simulink model "NewMY"  (Simulink 7.8)
settings: Solver=ode45  StartTime=0.0  StopTime=6  RelTol=1e-3
undefined symbols (not defined in the file): DiscIntNeverNeededParam
libraries: powerlib x8, simulink x4, powerlib_extras x2
settings Model: Creator=Meshkov  LastModifiedBy=suzdorf.vi  ModifiedComment=Meshkov -- Fri Mar 25 16:39:32 2011 -- Version 1.11
settings Model: ModifiedHistory=|
  | Meshkov -- Fri Mar 25 16:39:32 2011 -- Version 1.11
  | 
  | 
  | Meshkov -- Fri Mar 25 12:43:29 2011 -- Version 1.10
  | 
  | 
  | Meshkov -- Thu Mar 03 20:00:01 2011 -- Version 1.9
  | 
  | 
  | Meshkov -- Thu Mar 03 18:37:37 2011 -- Version 1.8
  | 
  | 
  | This model was created by Aleksander S. Meshkov on Feb 28. I don't khiw why I created that model...
  | so... may be i had wanted to write dissertation
settings DataIOCC: LimitDataPoints=off
settings DebuggingCC: FcnCallInpInsideContextMsg=Use local settings

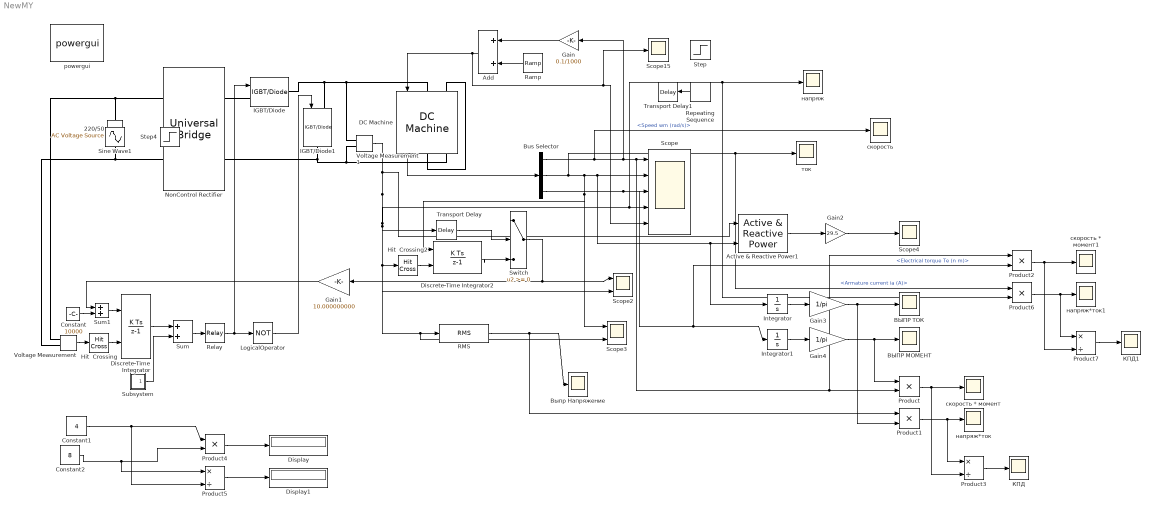
== system NewMY ==
  220/50 : powerlib/Electrical Sources/AC Voltage Source  Amplitude=220*sqrt(2)  Phase=0  Frequency=50  SampleTime=0  Measurements=None
  Active & Reactive Power1 : powerlib_extras/Measurements/Active & Reactive Power  f1=100
  Add : Sum
  Bus Selector : BusSelector  OutputSignals=Speed wm (rad/s),Armature current ia (A),Electrical torque Te (n m)
  Constant : Constant  Value=10000  SampleTime=0
  Constant1 : Constant  Value=4
  Constant2 : Constant  Value=8
  DC Machine : powerlib/Machines/DC Machine  PresetModel=No  MechanicalLoad=Torque TL  FieldType=Wound  ShowDetailedParameters=on  RLa="[ 7.061  0.058]"  RLf="[ 12.939  0.531]"  Laf=0.0098  MachineConstant=Torque constant (N.m/A)  Ke=1.8  Kt=1.8  J=0.21e-3  Bm=0  Tf=0  w0=1  Ifinit=-8.46539071434242e-022  TsPowergui=0  TsBlock=-1
      settings: AttributesFormatString=\n
  Discrete-Time Integrator : DiscreteIntegrator  gainval=1  ExternalReset=rising  SampleTime=2e-005  ICPrevOutput=DiscIntNeverNeededParam  ICPrevScaledInput=DiscIntNeverNeededParam
  Discrete-Time Integrator2 : DiscreteIntegrator  gainval=1  ExternalReset=rising  SampleTime=2e-005  ICPrevOutput=DiscIntNeverNeededParam  ICPrevScaledInput=DiscIntNeverNeededParam
  Display : Display
  Display1 : Display
  Gain : Gain  Gain=0.1/1000
  Gain1 : Gain  Gain=10.000000000
  Gain2 : Gain  Gain=29.5
  Gain3 : Gain  Gain=1/pi
  Gain4 : Gain  Gain=1/pi
  Hit  Crossing : HitCross  SampleTime=2e-005
  Hit  Crossing2 : HitCross  SampleTime=2e-005
  IGBT/Diode : powerlib/Power Electronics/IGBT//Diode  Ron=1e-3  Rs=1e5  Cs=inf  Measurements=off
  IGBT/Diode1 : powerlib/Power Electronics/IGBT//Diode  Ron=1e-3  Rs=1e5  Cs=inf  Measurements=off
  Integrator : Integrator
  Integrator1 : Integrator
  LogicalOperator : Logic  Operator=NOT  AllPortsSameDT=off  OutDataTypeStr=boolean
  NonControl Rectifier : powerlib/Power Electronics/Universal Bridge  Arms=2  SnubberResistance=1e5  SnubberCapacitance=inf  Device=Diodes  Ron=1e-3  Lon=0  ForwardVoltages="[  0  0  ]"  ForwardVoltage=0  GTOparameters=[ 10e-6 , 20e-6 ]  IGBTparameters=[ 1e-6 , 2e-6 ]  Measurements=Device currents  Measurements_2=None  converterType=Rectifier
  Product{,1..2,4,6} (5 alike) : Product  RndMeth=Zero
  Product3 : Product  Inputs=*/  RndMeth=Zero
  Product5 : Product  Inputs=*/  SaturateOnIntegerOverflow=on  RndMeth=Zero
  Product7 : Product  Inputs=*/  RndMeth=Zero
  RMS : powerlib_extras/Measurements/RMS  f1=100
  Ramp : simulink/Sources/Ramp  slope=-0.2  start=3  X0=0
  Relay : Relay  OnSwitchValue=0.1  OffSwitchValue=-0.1  OutDataTypeStr=Inherit: Inherit via back propagation
  Repeating Sequence : simulink/Sources/Repeating Sequence  rep_seq_t=[0 1]  rep_seq_y=[0 0.35]
  Scope : Scope  NumInputPorts=5
      settings: YMin=649.5~7.1~0.49~-50~0.5818  YMax=652~7.9~0.61~350~0.5827
  Scope15 : Scope
      settings: YMin=0  YMax=0.02  SaveName=Mc
  Scope2 : Scope  NumInputPorts=2
      settings: YMin=0~0  YMax=0.02~1  SaveName=current
  Scope3 : Scope  NumInputPorts=2
      settings: YMin=0~0  YMax=0.02~1  SaveName=current1
  Scope4 : Scope
      settings: YMin=0  YMax=0.02  SaveName=Mc1
  Step : Step  Time=4  After=0.252  SampleTime=0
  Subsystem : Subsystem
      mask Display: port_label('output', 1, '-C-')
  Sum : Sum  SaturateOnIntegerOverflow=on  InputSameDT=on  OutDataTypeStr=Inherit: Same as first input
  Sum1 : Sum  SaturateOnIntegerOverflow=on  InputSameDT=on  OutDataTypeStr=Inherit: Same as first input
  Switch : Switch  OutDataTypeStr=double  ZeroCross=off
  Transport Delay : TransportDelay  DelayTime=0.00003
  Transport Delay1 : TransportDelay  DelayTime=3
  Voltage Measurement : powerlib/Measurements/Voltage Measurement  PhasorSimulation=off  OutputType=Complex  PSBequivalent=0
  Voltage Measurement1 : powerlib/Measurements/Voltage Measurement  PhasorSimulation=off  OutputType=Complex  PSBequivalent=0
  powergui : powerlib/powergui  Priority=1  SimulationMode=Continuous  SolverType=Tustin  SampleTime=50e-6  frequency=60  SPID=on  DisableSnubberDevices=off  DisableRonSwitches=off  DisableVfSwitches=on  SwTol=0  Interpol=off  DisplayEquations=off  FunctionMessages=off  frequencyindice=50  Pbase=100e6  ErrMax=1e-4  Iterations=50  UnitsV=kV  UnitsW=MW  echomessages=off  HookPort=off  EnableUseOfTLC=off  x0status=blocks  RestoreLinks=warning  ResistiveCurrentMeasurement=off  Frange=[0:2:500]  Ylog=off  Xlog=on  ShowGrid=off  save=off  variable=ZData  structure=rmsU  ZoomFFT=off  StartTime=0.0  cycles=1  DisplayStyle=1  fundamental=60  FreqAxis=off  MaxFrequency=1000  frequencyindicesteady=1  RmsSteady=1  display=off  Ts=0  methode=off
  ВЫПР МОМЕНТ : Scope
      settings: YMin=0  YMax=0.02  SaveName=Mc6
  ВЫПР ТОК : Scope
      settings: YMin=0  YMax=0.02  SaveName=Mc5
  Выпр Напряжение : Scope
      settings: YMin=0  YMax=0.02  SaveName=rmsU
  КПД : Scope
      settings: YMin=0  YMax=0.02  SaveName=Mc9
  КПД1 : Scope
      settings: YMin=0  YMax=0.02  SaveName=Mc10
  напряж : Scope
      settings: YMin=0  YMax=0.02  SaveName=Mc2
  напряж*ток : Scope
      settings: YMin=0  YMax=0.02  SaveName=Mc8
  напряж*ток1 : Scope
      settings: YMin=0  YMax=0.02  SaveName=Mc11
  скорость : Scope
      settings: YMin=0  YMax=0.02  SaveName=Mc4
  скорость * момент : Scope
      settings: YMin=0  YMax=0.02  SaveName=Mc7
  скорость * момент1 : Scope
      settings: YMin=0  YMax=0.02  SaveName=Mc12
  ток : Scope
      settings: YMin=0  YMax=0.02  SaveName=Mc3
  Sine Wave1 : Sin  IOType=siggen  SampleTime=0
  Step4 : Step  IOType=siggen  SampleTime=0
  wires:
  Hit  Crossing/1 -> Discrete-Time Integrator/2
  Sum/1 -> Relay/1
  Add/1 -> DC Machine/1, Scope/5, Scope15/1
  Gain/1 -> Add/1
  Constant/1 -> Sum1/2
  Sum1/1 -> Discrete-Time Integrator/1
  Voltage Measurement/1 -> Hit  Crossing/1
  Hit  Crossing2/1 -> Discrete-Time Integrator2/2
  Discrete-Time Integrator2/1 -> Switch/3
  Switch/1 -> Gain1/1, Scope2/1
  Voltage Measurement1/1 -> Transport Delay/1, Hit  Crossing2/1, Scope2/2, Scope/4, напряж/1, Product6/2, RMS/1, Scope3/2, Active & Reactive Power1/1
  DC Machine/1 -> Bus Selector/1
  Bus Selector/2 -> Discrete-Time Integrator2/1, Scope3/1, Scope/2, Active & Reactive Power1/2, Integrator/1, ток/1, Product6/1  "<Armature current ia (A)>"
  Bus Selector/3 -> Scope/3, Integrator1/1, Product2/2  "<Electrical torque Te (n m)>"
  Bus Selector/1 -> Gain/1, Scope/1, Product/2, Product2/1, скорость/1  "<Speed wm (rad/s)>"
  Transport Delay/1 -> Switch/2
  Relay/1 -> LogicalOperator/1, IGBT/Diode/1
  Repeating Sequence/1 -> Transport Delay1/1
  LogicalOperator/1 -> IGBT/Diode1/1
  Gain1/1 -> Sum1/1
  RMS/1 -> Выпр Напряжение/1, Product1/1
  Ramp/1 -> Add/2
  Subsystem/1(Out1) -> Sum/2
  Discrete-Time Integrator/1 -> Sum/1
  Active & Reactive Power1/1 -> Gain2/1
  Gain2/1 -> Scope4/1
  Integrator/1 -> Gain3/1
  Gain3/1 -> ВЫПР ТОК/1, Product1/2
  Integrator1/1 -> Gain4/1
  Gain4/1 -> ВЫПР МОМЕНТ/1, Product/1
  Product/1 -> Product3/2, скорость * момент/1
  Product1/1 -> напряж*ток/1, Product3/1
  Product3/1 -> КПД/1
  Constant1/1 -> Product4/1, Product5/2
  Constant2/1 -> Product4/2, Product5/1
  Product5/1 -> Display1/1
  Product4/1 -> Display/1
  Product2/1 -> Product7/2, скорость * момент1/1
  Product6/1 -> напряж*ток1/1, Product7/1
  Product7/1 -> КПД1/1
  connections:
  IGBT/Diode/RConn1 -- IGBT/Diode1/LConn1 -- DC Machine/LConn1 -- Voltage Measurement1/LConn1
  DC Machine/RConn1 -- DC Machine/LConn2
  DC Machine/RConn2 -- NonControl Rectifier/RConn2 -- IGBT/Diode1/RConn1 -- Voltage Measurement1/LConn2
  NonControl Rectifier/RConn1 -- IGBT/Diode/LConn1
  220/50/RConn1 -- NonControl Rectifier/LConn1 -- Voltage Measurement/LConn1
  NonControl Rectifier/LConn2 -- 220/50/LConn1 -- Voltage Measurement/LConn2

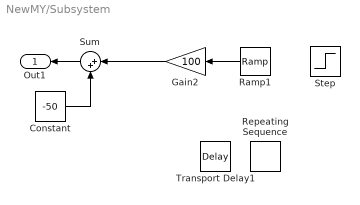
== system NewMY/Subsystem ==
  Constant : Constant  Value=-50
  Gain2 : Gain  Gain=100
  Ramp1 : simulink/Sources/Ramp  slope=0.115  start=3  X0=0
  Repeating Sequence : simulink/Sources/Repeating Sequence  rep_seq_t=[0 1]  rep_seq_y=[0 0.35]
  Step : Step  Time=4  After=0.252  SampleTime=0
  Sum : Sum  Inputs=|++
  Transport Delay1 : TransportDelay  DelayTime=3
  Out1 : Outport
  wires:
  Sum/1 -> Out1/1
  Constant/1 -> Sum/2
  Ramp1/1 -> Gain2/1
  Gain2/1 -> Sum/1
